simulink model "MyModel_Close_v1"  (R2018b)
settings: Solver=ode45  StartTime=0.0  StopTime=0.3  RelTol=1e-3
InitFcn:
  | tpwm = 0.0001;
  | K = 0.0604;
  | L1 = 0.00248;
  | L2 = -1.236e-7 * 40;
  | Td = 0;
  | kr = 50;
  | wc = 5;
  | speedref = 10;
  | L1 = 0.00248;
  | L2 = -1.239e-7 * 200;
libraries: powerlib x22, powerlib_meascontrol x12, powerlib_extras x5, simulink x2
settings Model: Creator=chenhao  LastModifiedBy=chenhao

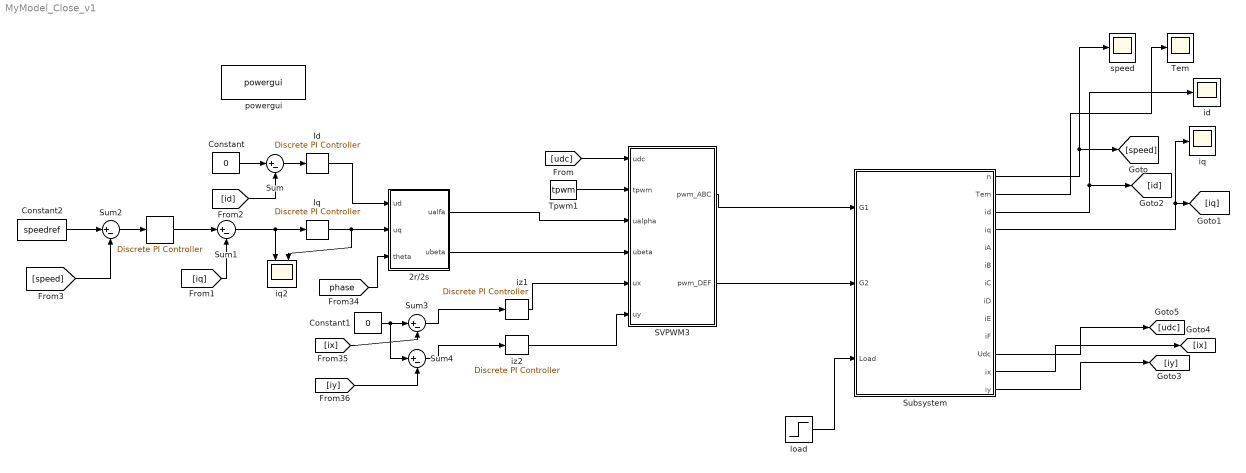
== system MyModel_Close_v1 ==
  "    " : powerlib_extras/Discrete  Control Blocks/Discrete PI Controller  Kp=1  Ki=80  Par_Limits=[50 -50]  Init=0  Ts=tpwm
  " Id" : powerlib_extras/Discrete  Control Blocks/Discrete PI Controller  Kp=3  Ki=120  Par_Limits=[300 -300]  Init=0  Ts=tpwm
  " Iq" : powerlib_extras/Discrete  Control Blocks/Discrete PI Controller  Kp=3  Ki=120  Par_Limits=[300 -300]  Init=0  Ts=tpwm
  " iz1" : powerlib_extras/Discrete  Control Blocks/Discrete PI Controller  Kp=10  Ki=100  Par_Limits=[300 -300]  Init=0  Ts=tpwm
  " iz2" : powerlib_extras/Discrete  Control Blocks/Discrete PI Controller  Kp=10  Ki=100  Par_Limits=[300 -300]  Init=0  Ts=tpwm
  2r/2s : Subsystem
  Constant : Constant  Value=0
  Constant1 : Constant  Value=0
  Constant2 : Constant  Value=speedref
  SVPWM3 : Subsystem
  Subsystem : Subsystem
  Sum{,1..4} (5 alike) : Sum  Inputs=|+-
  Tem : Scope
  Tpwm1 : Constant  Value=tpwm
  id : Scope
  iq : Scope
  iq2 : Scope  NumInputPorts=2
  load : Step  Time=0.1  After=5  SampleTime=0
  powergui : powerlib/powergui  Priority=1  SimulationMode=Discrete  SampleTime=5e-7  frequency=60  Iterations=50  frequencyindice=0  Pbase=100e6  ErrMax=1e-4  UnitsV=kV  UnitsW=MW  buscounter=0  FunctionMessages=off  echomessages=off  EnableUseOfTLC=off  CurrentSourceSwitches=off  DisableSnubberDevices=off  DisableRonSwitches=off  DisableVfSwitches=off  DisplayEquations=off  SolverType=Tustin  Interpol=off  ExternalGateDelay=off  methode=off  Ts=0  x0status=blocks  SPID=off  SwTol=0  HookPort=off  RestoreLinks=warning  ResistiveCurrentMeasurement=off  Frange=[0:2:500]  Ylog=off  Xlog=on  ShowGrid=off  save=off  variable=ZData  structure=Ia  ZoomFFT=on  StartTime=0.1  cycles=2  DisplayStyle=1  fundamental=2.5  FreqAxis=on  MaxFrequency=30  frequencyindicesteady=1  RmsSteady=1  display=off
  speed : Scope
  wires:
  SVPWM3/1(pwm_ABC) -> Subsystem/1(G1)
  " Iq"/1 -> iq2/2, 2r/2s/2(uq)
  " Id"/1 -> 2r/2s/1(ud)
  Sum/1 -> " Id"/1
  "    "/1 -> Sum1/1
  [id] -> Sum/2
  Sum1/1 -> iq2/1, " Iq"/1
  [iy] -> Sum4/2
  [speed] -> Sum2/2
  " iz2"/1 -> SVPWM3/6(uy)
  Tpwm1/1 -> SVPWM3/2(tpwm)
  [ix] -> Sum3/2
  Sum4/1 -> " iz2"/1
  Sum3/1 -> " iz1"/1
  Constant/1 -> Sum/1
  Sum2/1 -> "    "/1
  [phase] -> 2r/2s/3(theta)
  SVPWM3/2(pwm_DEF) -> Subsystem/2(G2)
  2r/2s/1(ualfa) -> SVPWM3/3(ualpha)
  [iq] -> Sum1/2
  2r/2s/2(ubeta) -> SVPWM3/4(ubeta)
  Constant1/1 -> Sum4/1, Sum3/1
  " iz1"/1 -> SVPWM3/5(ux)
  Constant2/1 -> Sum2/1
  Subsystem/1(n) -> speed/1, [speed]
  Subsystem/4(iq) -> iq/1, [iq]
  Subsystem/3(id) -> id/1, [id]
  Subsystem/12(ix) -> [ix]
  Subsystem/13("iy ") -> [iy]
  Subsystem/11(Udc) -> [udc]
  [udc] -> SVPWM3/1(udc)
  load/1 -> Subsystem/3(Load)
  Subsystem/2(Tem) -> Tem/1

== system MyModel_Close_v1/2r//2s ==
  ud : Inport
  uq : Inport  Port=2
  theta : Inport  Port=3
  Fcn : Fcn  Expr=u(1)*cos(u(3))-u(2)*sin(u(3))
  Fcn1 : Fcn  Expr=u(1)*sin(u(3))+u(2)*cos(u(3))
  Mux1 : Mux  Inputs=3
  ualfa : Outport
  ubeta : Outport  Port=2
  wires:
  theta/1 -> Mux1/3
  uq/1 -> Mux1/2
  ud/1 -> Mux1/1
  Fcn1/1 -> ubeta/1
  Fcn/1 -> ualfa/1
  Mux1/1 -> Fcn1/1, Fcn/1

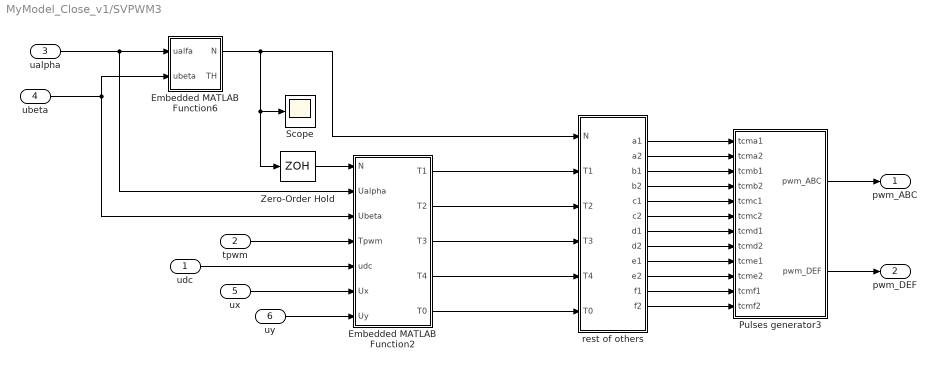
== system MyModel_Close_v1/SVPWM3 ==
  udc : Inport
  tpwm : Inport  Port=2
  ualpha : Inport  Port=3
  ubeta : Inport  Port=4
  ux : Inport  Port=5
  uy : Inport  Port=6
  Embedded MATLAB Function2 : MATLAB Function  TreatAsAtomicUnit=on
  Embedded MATLAB Function6 : MATLAB Function  TreatAsAtomicUnit=on
  Pulses generator3 : Subsystem
  Scope : Scope
  Zero-Order Hold : ZeroOrderHold  SampleTime=1e-4
  rest of others : MATLAB Function  TreatAsAtomicUnit=on
  pwm_ABC : Outport
  pwm_DEF : Outport  Port=2
  wires:
  udc/1 -> Embedded MATLAB Function2/5(udc)
  Embedded MATLAB Function2/4(T4) -> rest of others/5(T4)
  Embedded MATLAB Function2/1(T1) -> rest of others/2(T1)
  Pulses generator3/1(pwm_ABC) -> pwm_ABC/1
  Pulses generator3/2(pwm_DEF) -> pwm_DEF/1
  rest of others/12(f2) -> Pulses generator3/12(tcmf2)
  rest of others/11(f1) -> Pulses generator3/11(tcmf1)
  rest of others/10(e2) -> Pulses generator3/10(tcme2)
  rest of others/9(e1) -> Pulses generator3/9(tcme1)
  rest of others/8(d2) -> Pulses generator3/8(tcmd2)
  rest of others/7(d1) -> Pulses generator3/7(tcmd1)
  rest of others/6(c2) -> Pulses generator3/6(tcmc2)
  rest of others/5(c1) -> Pulses generator3/5(tcmc1)
  rest of others/4(b2) -> Pulses generator3/4(tcmb2)
  rest of others/3(b1) -> Pulses generator3/3(tcmb1)
  rest of others/2(a2) -> Pulses generator3/2(tcma2)
  rest of others/1(a1) -> Pulses generator3/1(tcma1)
  Embedded MATLAB Function2/2(T2) -> rest of others/3(T2)
  tpwm/1 -> Embedded MATLAB Function2/4(Tpwm)
  Embedded MATLAB Function2/5(T0) -> rest of others/6(T0)
  ualpha/1 -> Embedded MATLAB Function2/2(Ualpha), Embedded MATLAB Function6/1(ualfa)
  ubeta/1 -> Embedded MATLAB Function6/2(ubeta), Embedded MATLAB Function2/3(Ubeta)
  ux/1 -> Embedded MATLAB Function2/6(Ux)
  uy/1 -> Embedded MATLAB Function2/7(Uy)
  Embedded MATLAB Function2/3(T3) -> rest of others/4(T3)
  Zero-Order Hold/1 -> Embedded MATLAB Function2/1(N)
  Embedded MATLAB Function6/1(N) -> rest of others/1(N), Scope/1, Zero-Order Hold/1

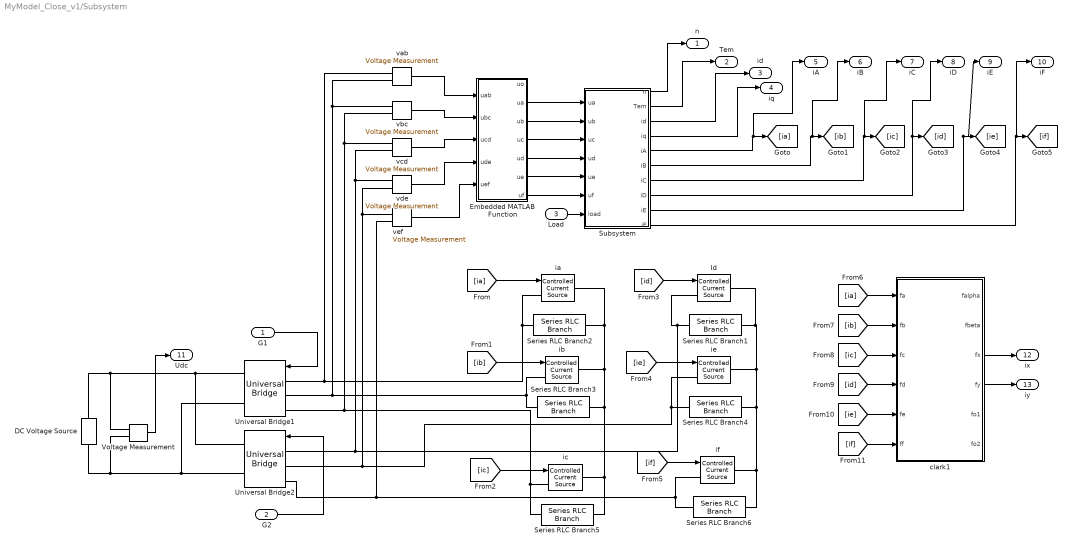
== system MyModel_Close_v1/Subsystem ==
  G1 : Inport
  G2 : Inport  Port=2
  Load : Inport  Port=3
  DC Voltage Source : powerlib/Electrical Sources/DC Voltage Source  Amplitude=100  Measurements=Voltage
  Embedded MATLAB Function : MATLAB Function  TreatAsAtomicUnit=on
  Id : powerlib/Electrical Sources/Controlled Current Source  Initialize=on  Source_Type=AC  Amplitude=0  Phase=0  Frequency=0  Measurements=None
  Series RLC Branch{1..6} (6 alike) : powerlib/Elements/Series RLC Branch  LConnTagsString=__new0  RConnTagsString=__new0  BranchType=R  Resistance=10e10  Inductance=10e-7  SetiL0=off  InitialCurrent=0  Capacitance=1e-6  Setx0=off  InitialVoltage=0  Measurements=None
  Subsystem : Subsystem
  Universal Bridge1 : powerlib/Power Electronics/Universal Bridge  Arms=3  SnubberResistance=1e5  SnubberCapacitance=inf  Device=IGBT / Diodes  Ron=1e-3  Lon=0  ForwardVoltages="[  0  0  ]"  ForwardVoltage=0  GTOparameters=[ 10e-6 , 20e-6 ]  IGBTparameters=[ 0 , 0 ]  Measurements=None  Measurements_2=None  converterType=Rectifier
  Universal Bridge2 : powerlib/Power Electronics/Universal Bridge  Arms=3  SnubberResistance=1e5  SnubberCapacitance=inf  Device=IGBT / Diodes  Ron=1e-3  Lon=0  ForwardVoltages="[  0  0  ]"  ForwardVoltage=0  GTOparameters=[ 10e-6 , 20e-6 ]  IGBTparameters=[ 0 , 0 ]  Measurements=None  Measurements_2=None  converterType=Rectifier
  Voltage Measurement : powerlib/Measurements/Voltage Measurement  PhasorSimulation=off  OutputType=Complex  PSBequivalent=0
  clark1 : MATLAB Function  TreatAsAtomicUnit=on
  ia : powerlib/Electrical Sources/Controlled Current Source  Initialize=on  Source_Type=AC  Amplitude=0  Phase=0  Frequency=0  Measurements=None
  ib : powerlib/Electrical Sources/Controlled Current Source  Initialize=on  Source_Type=AC  Amplitude=0  Phase=0  Frequency=0  Measurements=None
  ic : powerlib/Electrical Sources/Controlled Current Source  Initialize=on  Source_Type=AC  Amplitude=0  Phase=0  Frequency=0  Measurements=None
  ie : powerlib/Electrical Sources/Controlled Current Source  Initialize=on  Source_Type=AC  Amplitude=0  Phase=0  Frequency=0  Measurements=None
  if : powerlib/Electrical Sources/Controlled Current Source  Initialize=on  Source_Type=AC  Amplitude=0  Phase=0  Frequency=0  Measurements=None
  "vab " : powerlib/Measurements/Voltage Measurement  PhasorSimulation=off  OutputType=Complex  PSBequivalent=0
  vbc : powerlib/Measurements/Voltage Measurement  PhasorSimulation=off  OutputType=Complex  PSBequivalent=0
  vcd : powerlib/Measurements/Voltage Measurement  PhasorSimulation=off  OutputType=Complex  PSBequivalent=0
  vde : powerlib/Measurements/Voltage Measurement  PhasorSimulation=off  OutputType=Complex  PSBequivalent=0
  vef : powerlib/Measurements/Voltage Measurement  PhasorSimulation=off  OutputType=Complex  PSBequivalent=0
  n : Outport
  Tem : Outport  Port=2
  id : Outport  Port=3
  iq : Outport  Port=4
  iA : Outport  Port=5
  iB : Outport  Port=6
  iC : Outport  Port=7
  iD : Outport  Port=8
  iE : Outport  Port=9
  iF : Outport  Port=10
  Udc : Outport  Port=11
  ix : Outport  Port=12
  "iy " : Outport  Port=13
  wires:
  G1/1 -> Universal Bridge1/1
  G2/1 -> Universal Bridge2/1
  Voltage Measurement/1 -> Udc/1
  "vab "/1 -> Embedded MATLAB Function/1(uab)
  vbc/1 -> Embedded MATLAB Function/2(ubc)
  vcd/1 -> Embedded MATLAB Function/3(ucd)
  vde/1 -> Embedded MATLAB Function/4(ude)
  vef/1 -> Embedded MATLAB Function/5(uef)
  [ia] -> ia/1
  [ib] -> ib/1
  [ic] -> ic/1
  [id] -> Id/1
  [ie] -> ie/1
  [if] -> if/1
  [ia] -> clark1/1(fa)
  [ib] -> clark1/2(fb)
  [ic] -> clark1/3(fc)
  [id] -> clark1/4(fd)
  [ie] -> clark1/5(fe)
  [if] -> clark1/6(ff)
  clark1/3(fx) -> ix/1
  clark1/4(fy) -> "iy "/1
  Embedded MATLAB Function/6(ue) -> Subsystem/5(ue)
  Embedded MATLAB Function/2(ua) -> Subsystem/1(ua)
  Embedded MATLAB Function/3(ub) -> Subsystem/2(ub)
  Embedded MATLAB Function/4(uc) -> Subsystem/3(uc)
  Embedded MATLAB Function/5(ud) -> Subsystem/4(ud)
  Embedded MATLAB Function/7(uf) -> Subsystem/6(uf)
  Load/1 -> Subsystem/7(load)
  Subsystem/1(n) -> n/1
  Subsystem/2(Tem) -> Tem/1
  Subsystem/3(id) -> id/1
  Subsystem/4(iq) -> iq/1
  Subsystem/5(iA) -> iA/1, [ia]
  Subsystem/6(iB) -> iB/1, [ib]
  Subsystem/7(iC) -> iC/1, [ic]
  Subsystem/8(iD) -> iD/1, [id]
  Subsystem/9(iE) -> iE/1, [ie]
  Subsystem/10(iF) -> iF/1, [if]
  connections:
  Series RLC Branch4/LConn1 -- vef/LConn1 -- vde/LConn2 -- Universal Bridge2/LConn2 -- ie/LConn1
  Series RLC Branch6/LConn1 -- vef/LConn2 -- Universal Bridge2/LConn3 -- if/LConn1
  Universal Bridge1/RConn2 -- DC Voltage Source/LConn1 -- Voltage Measurement/LConn2 -- Universal Bridge2/RConn2
  DC Voltage Source/RConn1 -- Voltage Measurement/LConn1 -- Universal Bridge2/RConn1 -- Universal Bridge1/RConn1
  ia/LConn1 -- "vab "/LConn1 -- Universal Bridge1/LConn1 -- Series RLC Branch2/LConn1
  ib/LConn1 -- vbc/LConn1 -- "vab "/LConn2 -- Universal Bridge1/LConn2 -- Series RLC Branch3/LConn1
  ic/LConn1 -- vcd/LConn1 -- vbc/LConn2 -- Universal Bridge1/LConn3 -- Series RLC Branch5/LConn1
  Series RLC Branch2/RConn1 -- ia/RConn1 -- ib/RConn1 -- Series RLC Branch3/RConn1 -- ic/RConn1 -- Series RLC Branch5/RConn1
  Series RLC Branch1/RConn1 -- Id/RConn1 -- ie/RConn1 -- Series RLC Branch4/RConn1 -- if/RConn1 -- Series RLC Branch6/RConn1
  Universal Bridge2/LConn1 -- vde/LConn1 -- vcd/LConn2 -- Id/LConn1 -- Series RLC Branch1/LConn1

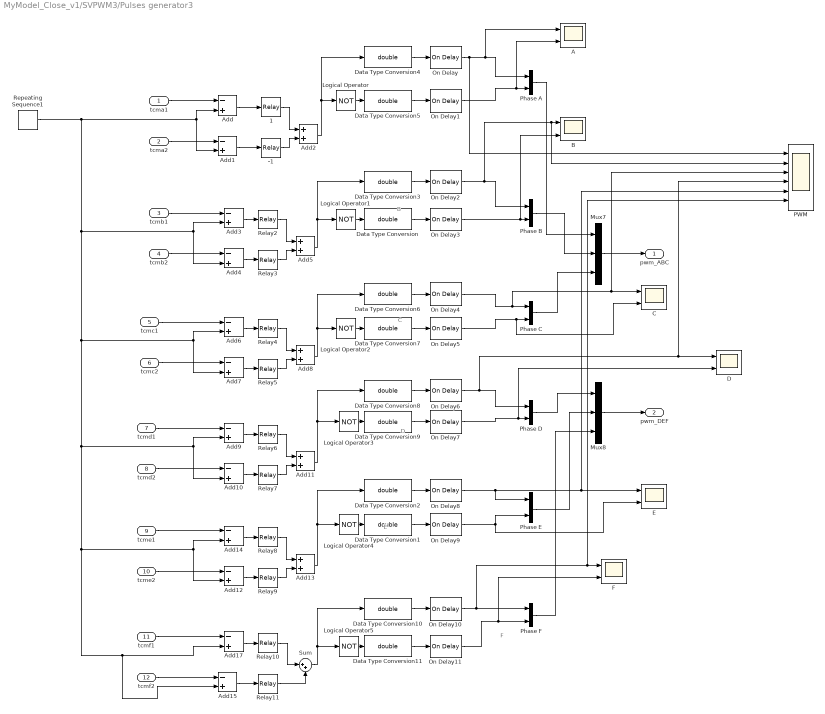
== system MyModel_Close_v1/SVPWM3/Pulses generator3 ==
  note: B
  note: C
  note: D
  note: E
  note: F
  tcma1 : Inport
  tcma2 : Inport  Port=2
  tcmb1 : Inport  Port=3
  tcmb2 : Inport  Port=4
  tcmc1 : Inport  Port=5
  tcmc2 : Inport  Port=6
  tcmd1 : Inport  Port=7
  tcmd2 : Inport  Port=8
  tcme1 : Inport  Port=9
  tcme2 : Inport  Port=10
  tcmf1 : Inport  Port=11
  tcmf2 : Inport  Port=12
  -1 : Relay  OnOutputValue=-1
  1 : Relay
  A : Scope  NumInputPorts=2
  Add{,1,3..4,6..7,9..10,12,14..15,17} (12 alike) : Sum  Inputs=-+
  Add{2,5,8,11,13} (5 alike) : Sum
  B : Scope  NumInputPorts=2
  C : Scope  NumInputPorts=2
  D : Scope  NumInputPorts=2
  Data Type Conversion{,1..11} (12 alike) : DataTypeConversion  OutDataTypeStr=double
  E : Scope  NumInputPorts=2
  F : Scope  NumInputPorts=2
  Logical Operator{,1..5} (6 alike) : Logic  Operator=NOT  AllPortsSameDT=off  OutDataTypeStr=boolean
  Mux7 : Mux  Inputs=3
  Mux8 : Mux  Inputs=3
  On Delay{,1..11} (12 alike) : powerlib_meascontrol/Logic/On Delay  DelayType=On delay  delay=Td  ic=0  Ts=0
      settings: SourceProductName=Simscape Power Systems
  PWM : Scope  NumInputPorts=6
  Phase A : Mux  Inputs=2
  Phase B : Mux  Inputs=2
  Phase C : Mux  Inputs=2
  Phase D : Mux  Inputs=2
  Phase E : Mux  Inputs=2
  Phase F : Mux  Inputs=2
  Relay{2,4,6,8,10} (5 alike) : Relay
  Relay{3,5,7,9,11} (5 alike) : Relay  OnOutputValue=-1
  Repeating Sequence1 : simulink/Sources/Repeating Sequence  rep_seq_t=[0 tpwm]  rep_seq_y=[0 tpwm]
  Sum : Sum  Inputs=|++
  pwm_ABC : Outport
  pwm_DEF : Outport  Port=2
  wires:
  On Delay11/1 -> F/2, Phase F/2
  Data Type Conversion11/1 -> On Delay11/1
  On Delay10/1 -> PWM/6, F/1, Phase F/1
  Data Type Conversion10/1 -> On Delay10/1
  On Delay9/1 -> E/2, Phase E/2
  Data Type Conversion1/1 -> On Delay9/1
  On Delay8/1 -> Phase E/1, PWM/5, E/1
  Data Type Conversion2/1 -> On Delay8/1
  On Delay7/1 -> D/2, Phase D/2
  Data Type Conversion9/1 -> On Delay7/1
  On Delay6/1 -> PWM/4, D/1, Phase D/1
  Data Type Conversion8/1 -> On Delay6/1
  On Delay5/1 -> C/2, Phase C/2
  Data Type Conversion7/1 -> On Delay5/1
  On Delay4/1 -> PWM/3, C/1, Phase C/1
  Data Type Conversion6/1 -> On Delay4/1
  On Delay2/1 -> PWM/2, B/1, Phase B/1
  On Delay3/1 -> B/2, Phase B/2
  Data Type Conversion/1 -> On Delay3/1
  Data Type Conversion3/1 -> On Delay2/1
  On Delay1/1 -> A/2, Phase A/2
  Data Type Conversion5/1 -> On Delay1/1
  On Delay/1 -> A/1, Phase A/1, PWM/1
  Data Type Conversion4/1 -> On Delay/1
  Logical Operator3/1 -> Data Type Conversion9/1
  Logical Operator2/1 -> Data Type Conversion7/1
  Logical Operator/1 -> Data Type Conversion5/1
  Logical Operator1/1 -> Data Type Conversion/1
  Logical Operator4/1 -> Data Type Conversion1/1
  Add5/1 -> Logical Operator1/1, Data Type Conversion3/1
  Add2/1 -> Logical Operator/1, Data Type Conversion4/1
  Mux8/1 -> pwm_DEF/1
  Mux7/1 -> pwm_ABC/1
  Sum/1 -> Logical Operator5/1, Data Type Conversion10/1
  Add13/1 -> Logical Operator4/1, Data Type Conversion2/1
  Add11/1 -> Logical Operator3/1, Data Type Conversion8/1
  Add8/1 -> Logical Operator2/1, Data Type Conversion6/1
  Logical Operator5/1 -> Data Type Conversion11/1
  tcmf2/1 -> Add15/1
  Relay11/1 -> Sum/2
  Relay10/1 -> Sum/1
  Add17/1 -> Relay10/1
  tcmf1/1 -> Add17/1
  tcme2/1 -> Add12/1
  Relay9/1 -> Add13/2
  Relay8/1 -> Add13/1
  Add12/1 -> Relay9/1
  Add14/1 -> Relay8/1
  tcme1/1 -> Add14/1
  tcmd2/1 -> Add10/1
  Relay7/1 -> Add11/2
  Relay6/1 -> Add11/1
  Add10/1 -> Relay7/1
  Add9/1 -> Relay6/1
  tcmd1/1 -> Add9/1
  tcmc2/1 -> Add7/1
  Relay5/1 -> Add8/2
  Relay4/1 -> Add8/1
  Add7/1 -> Relay5/1
  Add6/1 -> Relay4/1
  tcmb2/1 -> Add4/1
  Relay3/1 -> Add5/2
  Relay2/1 -> Add5/1
  Add4/1 -> Relay3/1
  Add3/1 -> Relay2/1
  tcma1/1 -> Add/1
  -1/1 -> Add2/2
  1/1 -> Add2/1
  Add1/1 -> -1/1
  Add/1 -> 1/1
  Repeating Sequence1/1 -> Add15/2, Add17/2, Add12/2, Add14/2, Add9/2, Add10/2, Add7/2, Add6/2, Add3/2, Add4/2, Add1/2, Add/2
  tcma2/1 -> Add1/1
  tcmb1/1 -> Add3/1
  tcmc1/1 -> Add6/1
  Add15/1 -> Relay11/1
  Phase A/1 -> Mux7/1
  Phase B/1 -> Mux7/2
  Phase C/1 -> Mux7/3
  Phase D/1 -> Mux8/1
  Phase E/1 -> Mux8/2
  Phase F/1 -> Mux8/3

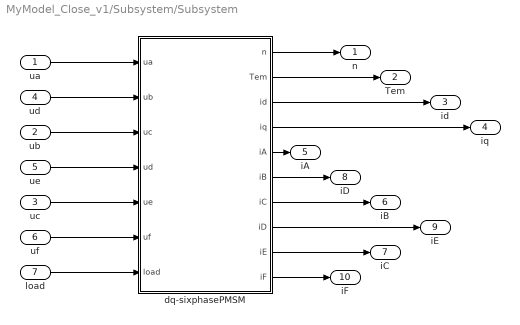
== system MyModel_Close_v1/Subsystem/Subsystem ==
  ua : Inport
  ub : Inport  Port=2
  uc : Inport  Port=3
  ud : Inport  Port=4
  ue : Inport  Port=5
  uf : Inport  Port=6
  load : Inport  Port=7
  dq-sixphasePMSM : Subsystem  mask{R=0.099, Ld=2.463342136542000e-03, Lq=2.473254136542000e-03, Lf=1.520747e-3, psi=0.0592, p=5, J=0.00174}
      mask prompts: R "Resistance (Om)"; Ld "d-inductance (H)"; Lq "q-inductance (H)"; Lf "Leak inductance (H)"; psi "flux (Wb)"; p "pole pairs"; J "inertia (kg*m^2)"
  n : Outport
  Tem : Outport  Port=2
  id : Outport  Port=3
  iq : Outport  Port=4
  iA : Outport  Port=5
  iB : Outport  Port=6
  iC : Outport  Port=7
  iD : Outport  Port=8
  iE : Outport  Port=9
  iF : Outport  Port=10
  wires:
  ua/1 -> dq-sixphasePMSM/1(ua)
  ub/1 -> dq-sixphasePMSM/3(uc)
  uc/1 -> dq-sixphasePMSM/5(ue)
  ud/1 -> dq-sixphasePMSM/2(ub)
  ue/1 -> dq-sixphasePMSM/4(ud)
  uf/1 -> dq-sixphasePMSM/6(uf)
  load/1 -> dq-sixphasePMSM/7(load)
  dq-sixphasePMSM/1(n) -> n/1
  dq-sixphasePMSM/2(Tem) -> Tem/1
  dq-sixphasePMSM/3(id) -> id/1
  dq-sixphasePMSM/4(iq) -> iq/1
  dq-sixphasePMSM/5(iA) -> iA/1
  dq-sixphasePMSM/6(iB) -> iD/1
  dq-sixphasePMSM/7(iC) -> iB/1
  dq-sixphasePMSM/8(iD) -> iE/1
  dq-sixphasePMSM/9(iE) -> iC/1
  dq-sixphasePMSM/10(iF) -> iF/1

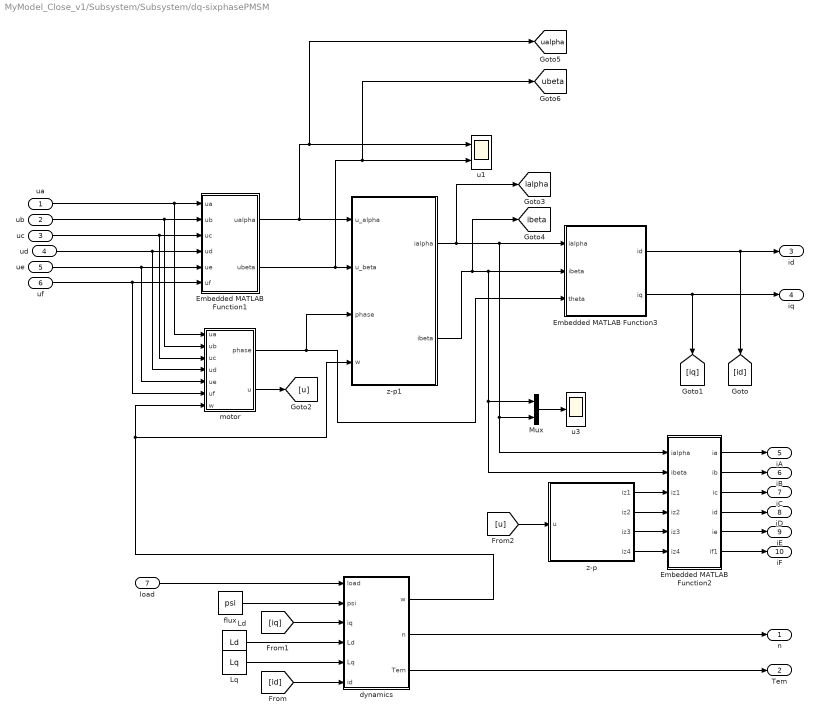
== system MyModel_Close_v1/Subsystem/Subsystem/dq-sixphasePMSM ==
  ua : Inport
  ub : Inport  Port=2
  uc : Inport  Port=3
  ud : Inport  Port=4
  ue : Inport  Port=5
  uf : Inport  Port=6
  load : Inport  Port=7
  Embedded MATLAB Function1 : MATLAB Function  TreatAsAtomicUnit=on
  Embedded MATLAB Function2 : MATLAB Function  TreatAsAtomicUnit=on
  Embedded MATLAB Function3 : MATLAB Function  TreatAsAtomicUnit=on
  Ld : Constant  Value=Ld
  Lq : Constant  Value=Lq
  Mux : Mux  Inputs=2
  dynamics : Subsystem
  flux : Constant  Value=psi
  motor : Subsystem
  u1 : Scope  NumInputPorts=2
  u3 : Scope
  z-p : Subsystem
  z-p1 : Subsystem
  n : Outport
  Tem : Outport  Port=2
  id : Outport  Port=3
  iq : Outport  Port=4
  iA : Outport  Port=5
  iB : Outport  Port=6
  iC : Outport  Port=7
  iD : Outport  Port=8
  iE : Outport  Port=9
  iF : Outport  Port=10
  tag scope: ialpha=global, ibeta=global, ualpha=global, ubeta=global
  wires:
  Embedded MATLAB Function2/3(ic) -> iC/1
  Embedded MATLAB Function2/5(ie) -> iE/1
  Embedded MATLAB Function2/4(id) -> iD/1
  Embedded MATLAB Function2/1(ia) -> iA/1
  Embedded MATLAB Function2/2(ib) -> iB/1
  Embedded MATLAB Function2/6(if1) -> iF/1
  ua/1 -> motor/1(ua), Embedded MATLAB Function1/1(ua)
  uc/1 -> motor/3(uc), Embedded MATLAB Function1/3(uc)
  ud/1 -> motor/4(ud), Embedded MATLAB Function1/4(ud)
  ue/1 -> motor/5(ue), Embedded MATLAB Function1/5(ue)
  uf/1 -> motor/6(uf), Embedded MATLAB Function1/6(uf)
  Ld/1 -> dynamics/4(Ld)
  Lq/1 -> dynamics/5(Lq)
  load/1 -> dynamics/1(load)
  flux/1 -> dynamics/2(psi)
  [id] -> dynamics/6(id)
  [iq] -> dynamics/3(iq)
  z-p/2(iz2) -> Embedded MATLAB Function2/4(iz2)
  z-p/1(iz1) -> Embedded MATLAB Function2/3(iz1)
  z-p/4(iz4) -> Embedded MATLAB Function2/6(iz4)
  z-p/3(iz3) -> Embedded MATLAB Function2/5(iz3)
  ub/1 -> motor/2(ub), Embedded MATLAB Function1/2(ub)
  [u] -> z-p/1(u)
  z-p1/1(ialpha) -> [ialpha], Mux/2, Embedded MATLAB Function2/1(ialpha), Embedded MATLAB Function3/1(ialpha)
  z-p1/2(ibeta) -> [ibeta], Mux/1, Embedded MATLAB Function2/2(ibeta), Embedded MATLAB Function3/2(ibeta)
  Embedded MATLAB Function3/1(id) -> [id], id/1
  Embedded MATLAB Function3/2(iq) -> iq/1, [iq]
  Mux/1 -> u3/1
  dynamics/1(w) -> z-p1/4(w), motor/7(w)
  dynamics/2(n) -> n/1
  dynamics/3(Tem) -> Tem/1
  motor/2(u) -> [u]
  motor/1(phase) -> Embedded MATLAB Function3/3(theta), z-p1/3(phase)
  Embedded MATLAB Function1/1(ualpha) -> [ualpha], u1/1, z-p1/1(u_alpha)
  Embedded MATLAB Function1/2(ubeta) -> [ubeta], u1/2, z-p1/2(u_beta)

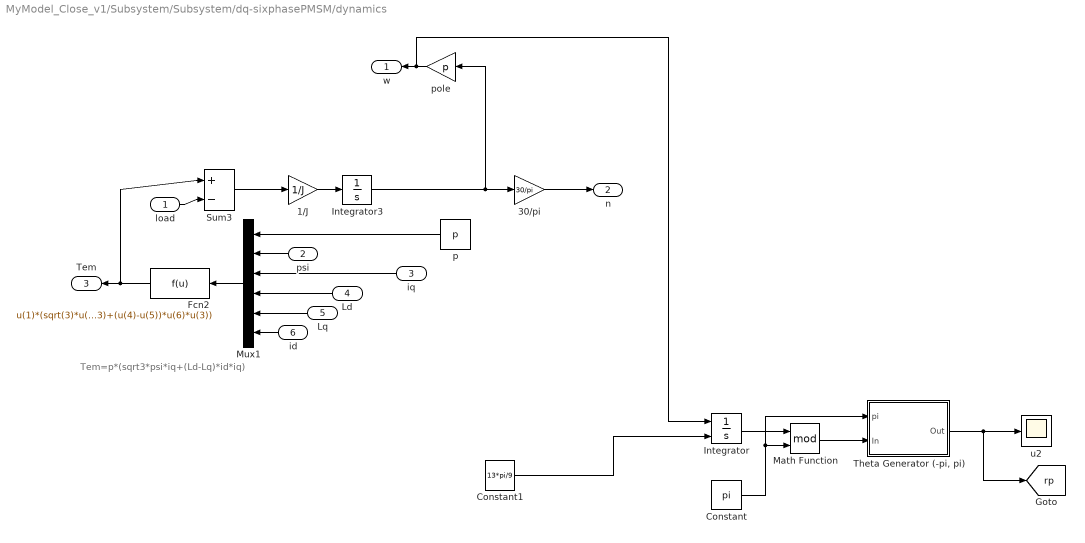
== system MyModel_Close_v1/Subsystem/Subsystem/dq-sixphasePMSM/dynamics ==
  note: Tem=p*(sqrt3*psi*iq+(Ld-Lq)*id*iq)
  load : Inport
  psi : Inport  Port=2
  iq : Inport  Port=3
  Ld : Inport  Port=4
  Lq : Inport  Port=5
  id : Inport  Port=6
  1/J : Gain  Gain=1/J  SaturateOnIntegerOverflow=on  OutDataTypeStr=Inherit: Same as input  ParamDataTypeStr=Inherit: Same as input
  30/pi : Gain  Gain=30/pi  SaturateOnIntegerOverflow=on  OutDataTypeStr=Inherit: Same as input  ParamDataTypeStr=Inherit: Same as input
  Constant : Constant  Value=pi
  Constant1 : Constant  Value=13*pi/9
  Fcn2 : Fcn  Expr=u(1)*(sqrt(3)*u(2)*u(3)+(u(4)-u(5))*u(6)*u(3))
  Integrator : Integrator  InitialConditionSource=external
  Integrator3 : Integrator
  Math Function : Math  Operator=mod  SaturateOnIntegerOverflow=on
  Mux1 : Mux  Inputs=6
  Sum3 : Sum  Inputs=|+-  SaturateOnIntegerOverflow=on
  "Theta Generator (-pi, pi)" : Subsystem
  p : Constant  Value=p
  pole : Gain  Gain=p  SaturateOnIntegerOverflow=on  OutDataTypeStr=Inherit: Same as input  ParamDataTypeStr=Inherit: Same as input
  u2 : Scope
  w : Outport
  n : Outport  Port=2
  Tem : Outport  Port=3
  tag scope: rp=global
  wires:
  p/1 -> Mux1/1
  Mux1/1 -> Fcn2/1
  Fcn2/1 -> Sum3/1, Tem/1
  Sum3/1 -> 1/J/1
  1/J/1 -> Integrator3/1
  Integrator3/1 -> 30/pi/1, pole/1
  psi/1 -> Mux1/2
  Ld/1 -> Mux1/4
  Lq/1 -> Mux1/5
  30/pi/1 -> n/1
  load/1 -> Sum3/2
  iq/1 -> Mux1/3
  id/1 -> Mux1/6
  pole/1 -> Integrator/1, w/1
  Integrator/1 -> Math Function/1
  Constant/1 -> Math Function/2, "Theta Generator (-pi, pi)"/1(pi)
  Math Function/1 -> "Theta Generator (-pi, pi)"/2(In)
  Constant1/1 -> Integrator/2
  "Theta Generator (-pi, pi)"/1(Out) -> [rp], u2/1

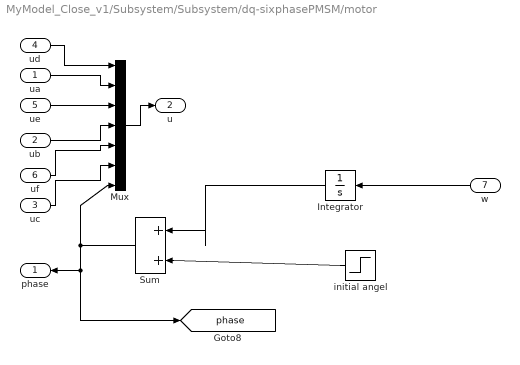
== system MyModel_Close_v1/Subsystem/Subsystem/dq-sixphasePMSM/motor ==
  ua : Inport
  ub : Inport  Port=2
  uc : Inport  Port=3
  ud : Inport  Port=4
  ue : Inport  Port=5
  uf : Inport  Port=6
  w : Inport  Port=7
  Integrator : Integrator
  Mux : Mux  Inputs=7
  Sum : Sum  Inputs=|++  SaturateOnIntegerOverflow=on
  initial angel : Step  Time=0  After=13*pi/9  SampleTime=0
  phase : Outport
  u : Outport  Port=2
  tag scope: phase=global
  wires:
  Sum/1 -> [phase], phase/1, Mux/7
  Integrator/1 -> Sum/1
  w/1 -> Integrator/1
  Mux/1 -> u/1
  ud/1 -> Mux/1
  ua/1 -> Mux/2
  ue/1 -> Mux/3
  ub/1 -> Mux/4
  uf/1 -> Mux/5
  uc/1 -> Mux/6
  initial angel/1 -> Sum/2

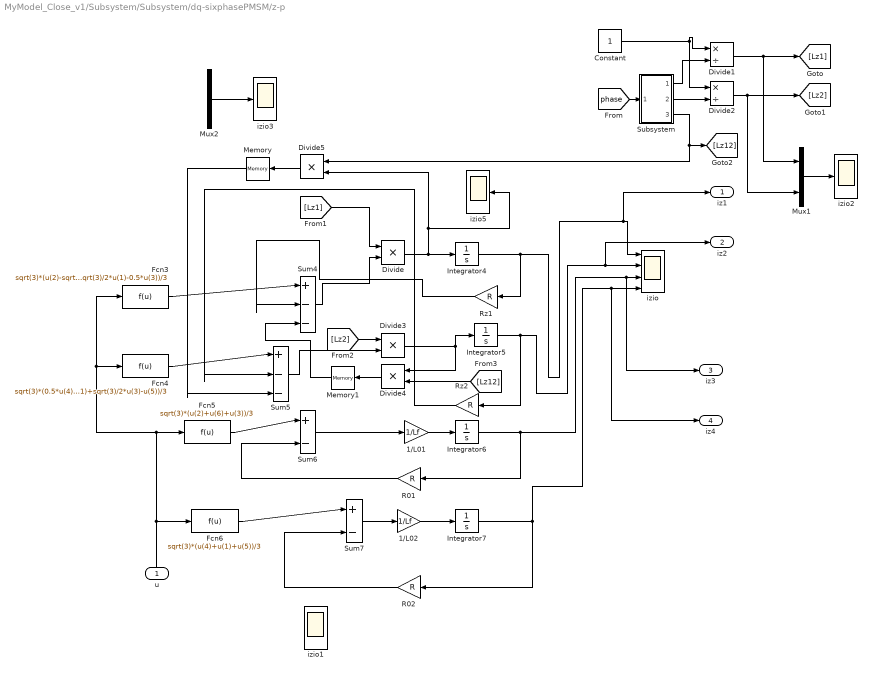
== system MyModel_Close_v1/Subsystem/Subsystem/dq-sixphasePMSM/z-p ==
  u : Inport
  1/L01 : Gain  Gain=1/Lf  SaturateOnIntegerOverflow=on  OutDataTypeStr=Inherit: Same as input  ParamDataTypeStr=Inherit: Same as input
  1/L02 : Gain  Gain=1/Lf  SaturateOnIntegerOverflow=on  OutDataTypeStr=Inherit: Same as input  ParamDataTypeStr=Inherit: Same as input
  Constant : Constant
  Divide{,3..5} (4 alike) : Product  Inputs=**
  Divide1 : Product  Inputs=*/
  Divide2 : Product  Inputs=*/
  Fcn3 : Fcn  Expr=sqrt(3)*(u(2)-sqrt(3)/2*u(4)-0.5*u(6)+sqrt(3)/2*u(1)-0.5*u(3))/3
  Fcn4 : Fcn  Expr=sqrt(3)*(0.5*u(4)-sqrt(3)/2*u(6)+0.5*u(1)+sqrt(3)/2*u(3)-u(5))/3
  Fcn5 : Fcn  Expr=sqrt(3)*(u(2)+u(6)+u(3))/3
  Fcn6 : Fcn  Expr=sqrt(3)*(u(4)+u(1)+u(5))/3
  Integrator{4..7} (4 alike) : Integrator
  Memory : Memory
  Memory1 : Memory
  Mux1 : Mux  Inputs=2
  Mux2 : Mux  Inputs=2
  R01 : Gain  Gain=R  SaturateOnIntegerOverflow=on  OutDataTypeStr=Inherit: Same as input  ParamDataTypeStr=Inherit: Same as input
  R02 : Gain  Gain=R  SaturateOnIntegerOverflow=on  OutDataTypeStr=Inherit: Same as input  ParamDataTypeStr=Inherit: Same as input
  Rz1 : Gain  Gain=R  SaturateOnIntegerOverflow=on  OutDataTypeStr=Inherit: Same as input  ParamDataTypeStr=Inherit: Same as input
  Rz2 : Gain  Gain=R  SaturateOnIntegerOverflow=on  OutDataTypeStr=Inherit: Same as input  ParamDataTypeStr=Inherit: Same as input
  Subsystem : Subsystem
  Sum4 : Sum  Inputs=|+--  SaturateOnIntegerOverflow=on
  Sum5 : Sum  Inputs=|+--  SaturateOnIntegerOverflow=on
  Sum6 : Sum  Inputs=|+-  SaturateOnIntegerOverflow=on
  Sum7 : Sum  Inputs=|+-  SaturateOnIntegerOverflow=on
  izio : Scope  NumInputPorts=4
  izio1 : Scope  NumInputPorts=4
  izio2 : Scope
  izio3 : Scope
  izio5 : Scope
  iz1 : Outport
  iz2 : Outport  Port=2
  iz3 : Outport  Port=3
  iz4 : Outport  Port=4
  wires:
  R02/1 -> Sum7/2
  R01/1 -> Sum6/2
  Rz2/1 -> Sum5/2
  Rz1/1 -> Sum4/2
  Integrator7/1 -> iz4/1, izio/4, R02/1
  1/L02/1 -> Integrator7/1
  Sum7/1 -> 1/L02/1
  Integrator6/1 -> iz3/1, izio/3, R01/1
  1/L01/1 -> Integrator6/1
  Sum6/1 -> 1/L01/1
  u/1 -> Fcn3/1, Fcn4/1, Fcn5/1, Fcn6/1
  [phase] -> Subsystem/1(Phase)
  Subsystem/1(Lz1) -> Divide1/2
  Divide1/1 -> Mux1/1, [Lz1]
  Constant/1 -> Divide1/1, Divide2/1
  Subsystem/2(Lz2) -> Divide2/2
  Divide2/1 -> Mux1/2, [Lz2]
  Mux1/1 -> izio2/1
  Sum4/1 -> Divide/2
  [Lz1] -> Divide/1
  Divide/1 -> izio5/1, Divide5/2, Integrator4/1
  Divide3/1 -> Integrator5/1, Divide4/1
  Sum5/1 -> Divide3/2
  [Lz2] -> Divide3/1
  Fcn5/1 -> Sum6/1
  Integrator5/1 -> Rz2/1, iz2/1, izio/2
  Integrator4/1 -> Rz1/1, iz1/1, izio/1
  Fcn4/1 -> Sum5/1
  Subsystem/3(Lz1z2) -> Divide5/1, [Lz12]
  Divide4/1 -> Memory1/1
  [Lz12] -> Divide4/2
  Divide5/1 -> Memory/1
  Memory1/1 -> Sum4/3
  Fcn6/1 -> Sum7/1
  Mux2/1 -> izio3/1
  Fcn3/1 -> Sum4/1
  Memory/1 -> Sum5/3

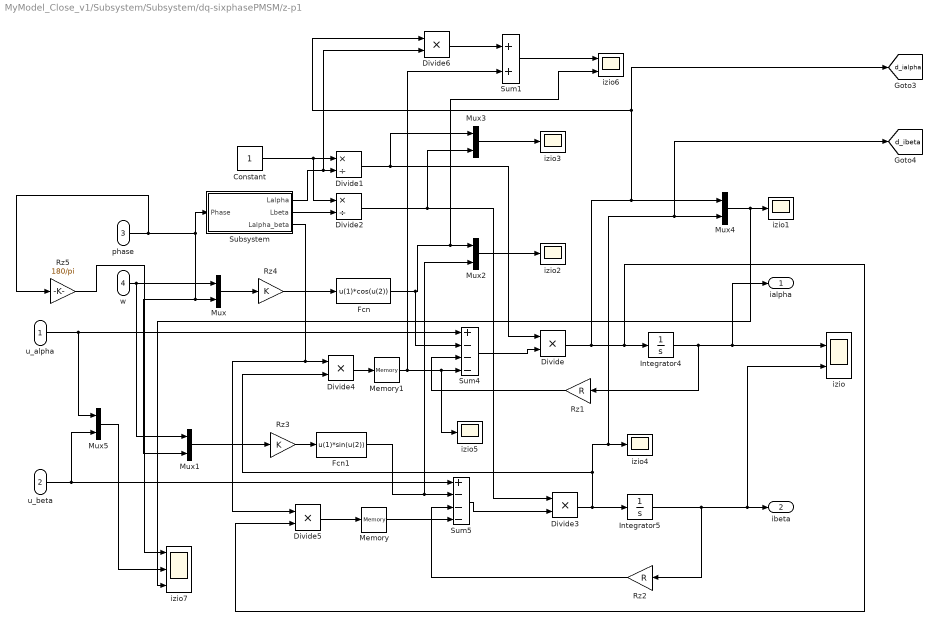
== system MyModel_Close_v1/Subsystem/Subsystem/dq-sixphasePMSM/z-p1 ==
  u_alpha : Inport
  u_beta : Inport  Port=2
  phase : Inport  Port=3
  w : Inport  Port=4
  Constant : Constant
  Divide{,3..6} (5 alike) : Product  Inputs=**
  Divide1 : Product  Inputs=*/
  Divide2 : Product  Inputs=*/
  Fcn : Fcn  Expr=u(1)*cos(u(2))
  Fcn1 : Fcn  Expr=u(1)*sin(u(2))
  Integrator4 : Integrator
  Integrator5 : Integrator
  Memory : Memory
  Memory1 : Memory
  Mux{,1..5} (6 alike) : Mux  Inputs=2
  Rz1 : Gain  Gain=R  SaturateOnIntegerOverflow=on  OutDataTypeStr=Inherit: Same as input  ParamDataTypeStr=Inherit: Same as input
  Rz2 : Gain  Gain=R  SaturateOnIntegerOverflow=on  OutDataTypeStr=Inherit: Same as input  ParamDataTypeStr=Inherit: Same as input
  Rz3 : Gain  Gain=K  SaturateOnIntegerOverflow=on  OutDataTypeStr=Inherit: Same as input  ParamDataTypeStr=Inherit: Same as input
  Rz4 : Gain  Gain=K  SaturateOnIntegerOverflow=on  OutDataTypeStr=Inherit: Same as input  ParamDataTypeStr=Inherit: Same as input
  Rz5 : Gain  Gain=180/pi  SaturateOnIntegerOverflow=on  OutDataTypeStr=Inherit: Same as input  ParamDataTypeStr=Inherit: Same as input
  Subsystem : Subsystem
  Sum1 : Sum  SaturateOnIntegerOverflow=on
  Sum4 : Sum  Inputs=+---  SaturateOnIntegerOverflow=on
  Sum5 : Sum  Inputs=+---  SaturateOnIntegerOverflow=on
  izio : Scope  NumInputPorts=2
  izio{1..5} (5 alike) : Scope
  izio6 : Scope  NumInputPorts=2
  izio7 : Scope  NumInputPorts=3
  ialpha : Outport
  ibeta : Outport  Port=2
  tag scope: d_ialpha=global, d_ibeta=global
  wires:
  phase/1 -> Rz5/1, Subsystem/1(Phase), Mux1/2, Mux/2
  Subsystem/1(Lalpha) -> Divide6/2, Divide1/2
  Constant/1 -> Divide1/1, Divide2/1
  Subsystem/2(Lbeta) -> Divide2/2
  Sum4/1 -> Divide/2
  Divide/1 -> Divide6/1, [d_ialpha], Mux4/1, Divide5/2, Integrator4/1
  Divide3/1 -> [d_ibeta], Mux4/2, izio4/1, Divide4/2, Integrator5/1
  Sum5/1 -> Divide3/2
  Integrator4/1 -> Rz1/1, ialpha/1, izio/1
  Rz1/1 -> Sum4/3
  Rz2/1 -> Sum5/3
  u_alpha/1 -> Mux5/1, Sum4/1
  u_beta/1 -> Mux5/2, Sum5/1
  Divide1/1 -> Mux3/1, Divide/1
  Divide2/1 -> Mux3/2, Divide3/1
  w/1 -> Mux/1, Mux1/1
  Mux/1 -> Rz4/1
  Fcn/1 -> Sum4/2, izio6/2, Mux2/1
  Fcn1/1 -> Mux2/2, Sum5/2
  Mux1/1 -> Rz3/1
  Divide4/1 -> Memory1/1
  Subsystem/3(Lalpha_beta) -> Divide4/1, Divide5/1
  Integrator5/1 -> Rz2/1, izio/2, ibeta/1
  Divide5/1 -> Memory/1
  Mux2/1 -> izio2/1
  Mux3/1 -> izio3/1
  Mux4/1 -> izio7/3, izio1/1
  Memory/1 -> Sum5/4
  Memory1/1 -> izio5/1, Sum4/4, Sum1/2
  Rz3/1 -> Fcn1/1
  Rz4/1 -> Fcn/1
  Divide6/1 -> Sum1/1
  Sum1/1 -> izio6/1
  Rz5/1 -> izio7/1
  Mux5/1 -> izio7/2

== system MyModel_Close_v1/Subsystem/Subsystem/dq-sixphasePMSM/dynamics/Theta Generator (-pi, pi) ==
  pi : Inport
  In : Inport  Port=2
  Compare To Constant : simulink/Logic and Bit Operations/Compare To Constant  relop=>  const=pi/2  OutDataTypeStr=uint8  ZeroCross=off
  Constant3 : Constant  Value=0
  Sum2 : Sum  Inputs=+-
  Switch : Switch  Threshold=0.5
  Out : Outport
  wires:
  Compare To Constant/1 -> Switch/2
  Switch/1 -> Sum2/2
  Constant3/1 -> Switch/3
  pi/1 -> Switch/1
  In/1 -> Sum2/1, Compare To Constant/1
  Sum2/1 -> Out/1

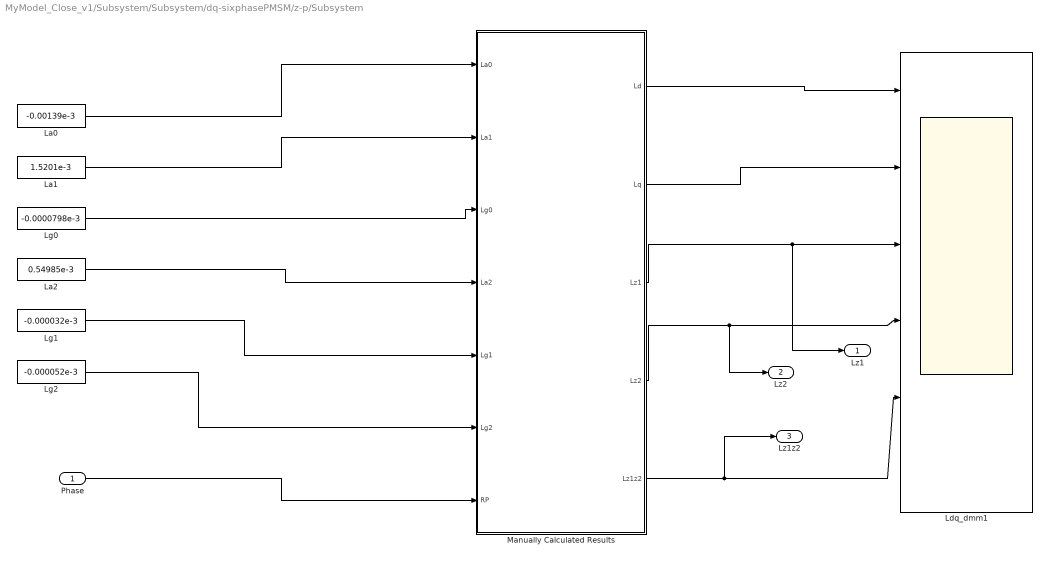
== system MyModel_Close_v1/Subsystem/Subsystem/dq-sixphasePMSM/z-p/Subsystem ==
  Phase : Inport
  La0 : Constant  Value=-0.00139e-3
  La1 : Constant  Value=1.5201e-3
  La2 : Constant  Value=0.54985e-3
  Ldq_dmm1 : Scope  NumInputPorts=6
  Lg0 : Constant  Value=-0.0000798e-3
  Lg1 : Constant  Value=-0.000032e-3
  Lg2 : Constant  Value=-0.000052e-3
  "Manually Calculated Results " : MATLAB Function  TreatAsAtomicUnit=on
  Lz1 : Outport
  Lz2 : Outport  Port=2
  Lz1z2 : Outport  Port=3
  wires:
  "Manually Calculated Results "/3(Lz1) -> Lz1/1, Ldq_dmm1/3
  Lg2/1 -> "Manually Calculated Results "/6(Lg2)
  Lg1/1 -> "Manually Calculated Results "/5(Lg1)
  "Manually Calculated Results "/2(Lq) -> Ldq_dmm1/2
  Lg0/1 -> "Manually Calculated Results "/3(Lg0)
  "Manually Calculated Results "/4(Lz2) -> Lz2/1, Ldq_dmm1/4
  "Manually Calculated Results "/1(Ld) -> Ldq_dmm1/1
  "Manually Calculated Results "/5(Lz1z2) -> Lz1z2/1, Ldq_dmm1/5
  La0/1 -> "Manually Calculated Results "/1(La0)
  La1/1 -> "Manually Calculated Results "/2(La1)
  La2/1 -> "Manually Calculated Results "/4(La2)
  Phase/1 -> "Manually Calculated Results "/7(RP)

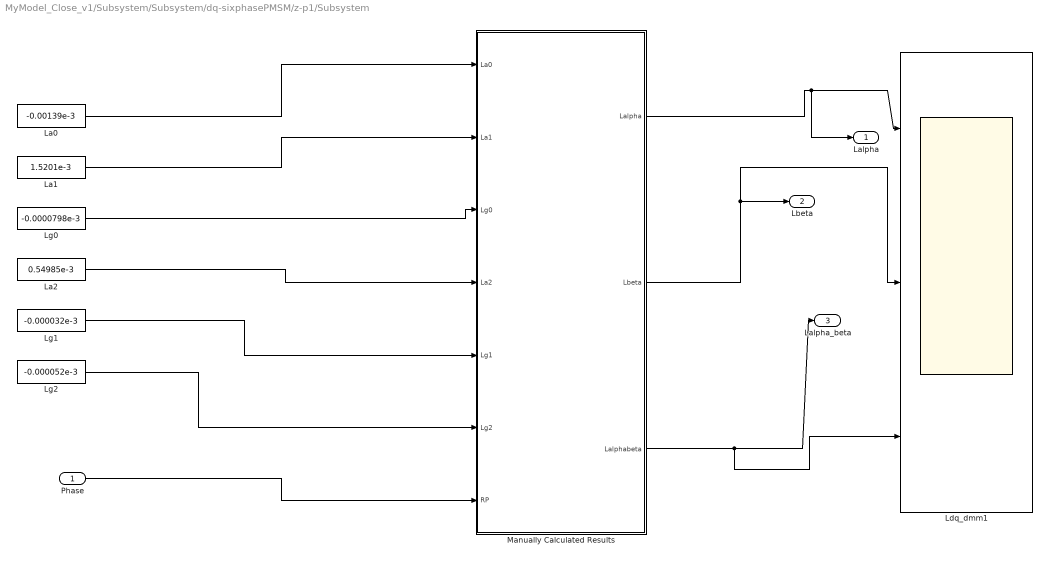
== system MyModel_Close_v1/Subsystem/Subsystem/dq-sixphasePMSM/z-p1/Subsystem ==
  Phase : Inport
  La0 : Constant  Value=-0.00139e-3
  La1 : Constant  Value=1.5201e-3
  La2 : Constant  Value=0.54985e-3
  Ldq_dmm1 : Scope  NumInputPorts=3
  Lg0 : Constant  Value=-0.0000798e-3
  Lg1 : Constant  Value=-0.000032e-3
  Lg2 : Constant  Value=-0.000052e-3
  "Manually Calculated Results " : MATLAB Function  TreatAsAtomicUnit=on
  Lalpha : Outport
  Lbeta : Outport  Port=2
  Lalpha_beta : Outport  Port=3
  wires:
  Lg2/1 -> "Manually Calculated Results "/6(Lg2)
  Lg1/1 -> "Manually Calculated Results "/5(Lg1)
  "Manually Calculated Results "/2(Lbeta) -> Ldq_dmm1/2, Lbeta/1
  Lg0/1 -> "Manually Calculated Results "/3(Lg0)
  "Manually Calculated Results "/1(Lalpha) -> Lalpha/1, Ldq_dmm1/1
  La0/1 -> "Manually Calculated Results "/1(La0)
  La1/1 -> "Manually Calculated Results "/2(La1)
  La2/1 -> "Manually Calculated Results "/4(La2)
  Phase/1 -> "Manually Calculated Results "/7(RP)
  "Manually Calculated Results "/3(Lalphabeta) -> Ldq_dmm1/3, Lalpha_beta/1

== matlab function MyModel_Close_v1/Subsystem/clark1 ==
  data: falpha output; fa input; fbeta output; fb input; fc input; fd input; fe input; fx output; fy output; fo1 output; fo2 output; ff input
function [falpha,fbeta,fx,fy,fo1,fo2] = clark(fa,fb,fc,fd,fe,ff)

T=1/sqrt(3)*[1,  (-1/2),    (-1/2),       sqrt(3)/2,  -sqrt(3)/2,  0;
       0,  sqrt(3)/2, (-sqrt(3)/2), 1/2,        1/2,        -1;
       1,  (-1/2),    (-1/2),       -sqrt(3)/2, sqrt(3)/2,   0;
       0,  -sqrt(3)/2,sqrt(3)/2,    1/2,        1/2,        -1;
       1,  1,         1,            0,          0,           0;
       0,  0,         0,            1,          1,           1];
X=[fa;fb;fc;fd;fe;ff];
Y=T*X;
falpha=Y(1);
fbeta=Y(2);
fx=Y(3);
fy=Y(4);
fo1=Y(5);
fo2=Y(6);
end

== matlab function MyModel_Close_v1/Subsystem/Embedded MATLAB Function ==
  data: uo output; uab input; ua output; ubc input; ucd input; ude input; uef input; ub output; uc output; ud output; ue output; uf output
function [uo,ua,ub,uc,ud,ue,uf] = fcn(uab,ubc,ucd,ude,uef)

%#codegen
uxx = [uab,ubc,ucd,ude,uef,0,0]';
T = [0 1 -1 0 0 0 0;
     0 0 1 -1 0 0 0;
     1 0 0 1 -1 0 0;
     0 0 0 0 1 -1 0;
     0 0 0 0 0 1 -1;
     0 1 1 1 0 0 0;
     0 0 0 0 1 1 1];
I = T \ uxx;
uo = I(1);
ua = I(2);
ub = I(3);
uc = I(4);
ud = I(5);
ue = I(6);
uf = I(7);

== matlab function MyModel_Close_v1/Subsystem/Subsystem/dq-sixphasePMSM/Embedded MATLAB Function1 ==
  data: ualpha output; ua input; ub input; uc input; ud input; ue input; uf input; ubeta output
function [ualpha,ubeta] = fcn(ua,ub,uc,ud,ue,uf)

%#eml
uxx=[ua,ub,uc,ud,ue,uf]';
T=1/sqrt(3)*[1 sqrt(3)/2 -1/2 -sqrt(3)/2 -1/2 0;
    0 1/2 sqrt(3)/2 1/2 -sqrt(3)/2 -1;
    1 -sqrt(3)/2 -1/2 sqrt(3)/2 -1/2 0;
    0 1/2 -sqrt(3)/2 1/2 sqrt(3)/2 -1;
    1 0 1 0 1 0;
    0 1 0 1 0 1];
I=T*uxx;
ualpha=I(1);
ubeta=I(2);

== matlab function MyModel_Close_v1/Subsystem/Subsystem/dq-sixphasePMSM/Embedded MATLAB Function2 ==
  data: ia output; ialpha input; ibeta input; iz1 input; iz2 input; iz3 input; iz4 input; ib output; ic output; id output; ie output; if1 output
function [ia,ib,ic,id,ie,if1] = fcn(ialpha,ibeta,iz1,iz2,iz3,iz4)

%#eml
uxx=[ialpha,ibeta,iz1,iz2,iz3,iz4]';
T=1/sqrt(3)*[1 sqrt(3)/2 -1/2 -sqrt(3)/2 -1/2 0;
    0 1/2 sqrt(3)/2 1/2 -sqrt(3)/2 -1;
    1 -sqrt(3)/2 -1/2 sqrt(3)/2 -1/2 0;
    0 1/2 -sqrt(3)/2 1/2 sqrt(3)/2 -1;
    1 0 1 0 1 0;
    0 1 0 1 0 1];
I=inv(T)*uxx;
ia=I(1);
ib=I(2);
ic=I(3);
id=I(4);
ie=I(5);
if1=I(6);

== matlab function MyModel_Close_v1/Subsystem/Subsystem/dq-sixphasePMSM/Embedded MATLAB Function3 ==
  data: ialpha input; id output; iq output; ibeta input; theta input
function [id,iq] = fcn(ialpha,ibeta,theta)

%#eml
uxx=[ialpha,ibeta]';
T=[cos(theta),-sin(theta);sin(theta),cos(theta)];
I=inv(T)*uxx;
id=I(1);
iq=I(2);

== matlab function MyModel_Close_v1/Subsystem/Subsystem/dq-sixphasePMSM/z-p/Subsystem/Manually Calculated Results  ==
  data: La0 input; Ld output; La1 input; Lg0 input; La2 input; Lg1 input; Lg2 input; RP input; Lq output; Lz1 output; Lz2 output; Lz1z2 output
function [Ld,Lq,Lz1,Lz2,Lz1z2] = fcn(La0,La1,Lg0,La2,Lg1,Lg2,RP)
%#codegen
Ld=3*La0+La1+sqrt(3)*La2+40*(1/2*Lg0+Lg1+Lg2);
Lq=3*La0+sqrt(3)*La2+La1-40*(1/2*Lg0+Lg1+Lg2);
Lz1=La1+cos(2*RP)*40*(1/2*Lg0-Lg1+Lg2)-sqrt(3)*La2;
Lz2=La1-cos(2*RP)*40*(1/2*Lg0-Lg1+Lg2)-sqrt(3)*La2;
Lz1z2=-sin(2*RP)*40*(1/2*Lg0-Lg1+Lg2);

== matlab function MyModel_Close_v1/Subsystem/Subsystem/dq-sixphasePMSM/z-p1/Subsystem/Manually Calculated Results  ==
  data: La0 input; Lalpha output; La1 input; Lg0 input; La2 input; Lg1 input; Lg2 input; RP input; Lbeta output; Lalphabeta output
function [Lalpha,Lbeta,Lalphabeta] = fcn(La0,La1,Lg0,La2,Lg1,Lg2,RP)
%#codegen
Lalpha=3*La0+La1+sqrt(3)*La2+40*(1/2*Lg0+Lg1+Lg2)*cos(2*RP);
Lbeta=3*La0+sqrt(3)*La2+La1-40*(1/2*Lg0+Lg1+Lg2)*cos(2*RP);
Lalphabeta=40*(1/2*Lg0+Lg1+Lg2)*sin(2*RP);

== matlab function MyModel_Close_v1/SVPWM3/Embedded MATLAB Function2 ==
  data: N input; T1 output; Ualpha input; Ubeta input; Tpwm input; T2 output; T3 output; T4 output; T0 output; udc input; Ux input; Uy input
function [T1, T2, T3, T4, T0] = fcn(N, Ualpha, Ubeta, Tpwm, udc, Ux,Uy)

m=sqrt(3)/2+1/2*1i;

%等功率clarke反变换
ab44=1/sqrt(3)*udc*[1,m^4,m^8,m,m^5,m^9]*[1;0;0;1;0;0];
xy44=1/sqrt(3)*udc*[1,m^8,m^4,m^5,m,m^9]*[1;0;0;1;0;0];

ab64=1/sqrt(3)*udc*[1,m^4,m^8,m,m^5,m^9]*[1;1;0;1;0;0];
xy64=1/sqrt(3)*udc*[1,m^8,m^4,m^5,m,m^9]*[1;1;0;1;0;0];
        
ab66=1/sqrt(3)*udc*[1,m^4,m^8,m,m^5,m^9]*[1;1;0;1;1;0];
xy66=1/sqrt(3)*udc*[1,m^8,m^4,m^5,m,m^9]*[1;1;0;1;1;0];

ab26=1/sqrt(3)*udc*[1,m^4,m^8,m,m^5,m^9]*[0;1;0;1;1;0];
xy26=1/sqrt(3)*udc*[1,m^8,m^4,m^5,m,m^9]*[0;1;0;1;1;0];

ab22=1/sqrt(3)*udc*[1,m^4,m^8,m,m^5,m^9]*[0;1;0;0;1;0];
xy22=1/sqrt(3)*udc*[1,m^8,m^4,m^5,m,m^9]*[0;1;0;0;1;0];

ab32=1/sqrt(3)*udc*[1,m^4,m^8,m,m^5,m^9]*[0;1;1;0;1;0];
xy32=1/sqrt(3)*udc*[1,m^8,m^4,m^5,m,m^9]*[0;1;1;0;1;0];

ab33=1/sqrt(3)*udc*[1,m^4,m^8,m,m^5,m^9]*[0;1;1;0;1;1];
xy33=1/sqrt(3)*udc*[1,m^8,m^4,m^5,m,m^9]*[0;1;1;0;1;1];

ab13=1/sqrt(3)*udc*[1,m^4,m^8,m,m^5,m^9]*[0;0;1;0;1;1];
xy13=1/sqrt(3)*udc*[1,m^8,m^4,m^5,m,m^9]*[0;0;1;0;1;1];

ab11=1/sqrt(3)*udc*[1,m^4,m^8,m,m^5,m^9]*[0;0;1;0;0;1];
xy11=1/sqrt(3)*udc*[1,m^8,m^4,m^5,m,m^9]*[0;0;1;0;0;1];

ab51=1/sqrt(3)*udc*[1,m^4,m^8,m,m^5,m^9]*[1;0;1;0;0;1];
xy51=1/sqrt(3)*udc*[1,m^8,m^4,m^5,m,m^9]*[1;0;1;0;0;1];

ab55=1/sqrt(3)*udc*[1,m^4,m^8,m,m^5,m^9]*[1;0;1;1;0;1];
xy55=1/sqrt(3)*udc*[1,m^8,m^4,m^5,m,m^9]*[1;0;1;1;0;1];

ab45=1/sqrt(3)*udc*[1,m^4,m^8,m,m^5,m^9]*[1;0;0;1;0;1];
xy45=1/sqrt(3)*udc*[1,m^8,m^4,m^5,m,m^9]*[1;0;0;1;0;1];

switch N
    case 1
        X=[real(ab55),real(ab45),real(ab44),real(ab64);
           imag(ab55),imag(ab45),imag(ab44),imag(ab64);
           real(xy55),real(xy45),real(xy44),real(xy64);
           imag(xy55),imag(xy45),imag(xy44),imag(xy64)];

    case 2
        X=[real(ab45),real(ab44),real(ab64),real(ab66);
           imag(ab45),imag(ab44),imag(ab64),imag(ab66);
           real(xy45),real(xy44),real(xy64),real(xy66);
           imag(xy45),imag(xy44),imag(xy64),imag(xy66)];

    case 3
        X=[real(ab44),real(ab64),real(ab66),real(ab26);
           imag(ab44),imag(ab64),imag(ab66),imag(ab26);
           real(xy44),real(xy64),real(xy66),real(xy26);
           imag(xy44),imag(xy64),imag(xy66),imag(xy26)];

    case 4
        X=[real(ab64),real(ab66),real(ab26),real(ab22);
           imag(ab64),imag(ab66),imag(ab26),imag(ab22);
           real(xy64),real(xy66),real(xy26),real(xy22);
           imag(xy64),imag(xy66),imag(xy26),imag(xy22)];

    case 5
        X=[real(ab66),real(ab26),real(ab22),real(ab32);
           imag(ab66),imag(ab26),imag(ab22),imag(ab32);
           real(xy66),real(xy26),real(xy22),real(xy32);
           imag(xy66),imag(xy26),imag(xy22),imag(xy32)];

    case 6
        X=[real(ab26),real(ab22),real(ab32),real(ab33);
           imag(ab26),imag(ab22),imag(ab32),imag(ab33);
           real(xy26),real(xy22),real(xy32),real(xy33);
           imag(xy26),imag(xy22),imag(xy32),imag(xy33)];

    case 7
        X=[real(ab22),real(ab32),real(ab33),real(ab13);
           imag(ab22),imag(ab32),imag(ab33),imag(ab13);
           real(xy22),real(xy32),real(xy33),real(xy13);
           imag(xy22),imag(xy32),imag(xy33),imag(xy13)];

    case 8
        X=[real(ab32),real(ab33),real(ab13),real(ab11);
           imag(ab32),imag(ab33),imag(ab13),imag(ab11);
           real(xy32),real(xy33),real(xy13),real(xy11);
           imag(xy32),imag(xy33),imag(xy13),imag(xy11)];

    case 9
        X=[real(ab33),real(ab13),real(ab11),real(ab51);
           imag(ab33),imag(ab13),imag(ab11),imag(ab51);
           real(xy33),real(xy13),real(xy11),real(xy51);
           imag(xy33),imag(xy13),imag(xy11),imag(xy51)];

    case 10
        X=[real(ab13),real(ab11),real(ab51),real(ab55);
           imag(ab13),imag(ab11),imag(ab51),imag(ab55);
           real(xy13),real(xy11),real(xy51),real(xy55);
           imag(xy13),imag(xy11),imag(xy51),imag(xy55)];

    case 11
        X=[real(ab11),real(ab51),real(ab55),real(ab45);
           imag(ab11),imag(ab51),imag(ab55),imag(ab45);
           real(xy11),real(xy51),real(xy55),real(xy45);
           imag(xy11),imag(xy51),imag(xy55),imag(xy45)];

    case 12
        X=[real(ab51),real(ab55),real(ab45),real(ab44);
           imag(ab51),imag(ab55),imag(ab45),imag(ab44);
           real(xy51),real(xy55),real(xy45),real(xy44);
           imag(xy51),imag(xy55),imag(xy45),imag(xy44)];

    otherwise
        X=[0,0,0,0;
           0,0,0,0;
           0,0,0,0;
           0,0,0,0];

end
Y=[Ualpha;Ubeta;Ux;Uy]*Tpwm;
T = X \ Y;

T1=T(1);
if T1<15e-6
    T1=15e-6;
end 
T2=T(2);
if T2<15e-6
    T2=15e-6;
end 
T3=T(3);
if T3<1e-6
    T3=1e-6;
end 
T4=T(4);
if T4<1e-6
    T4=1e-6;
end

% T1=T(1);
% T2=T(2);
% T3=T(3);
% T4=T(4);

Tsum=T1+T2+T3+T4;
if Tsum>Tpwm
    T1=T1*Tpwm/Tsum;
    T2=T2*Tpwm/Tsum;
    T3=T3*Tpwm/Tsum;
    T4=T4*Tpwm/Tsum;
end
T0=Tpwm-T1-T2-T3-T4;
end

== matlab function MyModel_Close_v1/SVPWM3/Embedded MATLAB Function6 ==
  data: N output; ualfa input; ubeta input; TH output
function [N,TH] = fcn(ualfa,ubeta)

%#xsxx
[TH,R] = cart2pol(ualfa,ubeta);
if TH<0
    TH=TH+2*pi;
end
N=floor((TH+pi/12)/(pi/6))+1;
if N==13
    N=1;
end;

== matlab function MyModel_Close_v1/SVPWM3/rest of others ==
  data: N input; T1 input; T2 input; T3 input; T4 input; T0 input; a1 output; a2 output; b1 output; b2 output; c1 output; c2 output; d1 output; d2 output; e1 output; e2 output; f1 output; f2 output
function [a1,a2,b1,b2,c1,c2,d1,d2,e1,e2,f1,f2] = fcn(N,T1,T2,T3,T4,T0)

%#xsxx
Ta=T0/4;
Tb=Ta+T2;
Tc=Tb+T1;
Td=Tc+T0/2;
Te=Td+T4;
Tf=Te+T3;

Ta1=T0/4;
Tb1=Ta1+T1;
Tc1=Tb1+T2;
Td1=Tc1+T0/2;
Te1=Td1+T3;
Tf1=Te1+T4;

%a1:phase A CMPA
%a2:phase A CMPB

a1 = 0;
a2 = 0;
b1 = 0;
b2 = 0;
c1 = 0;
c2 = 0;
d1 = 0;
d2 = 0;
e1 = 0;
e2 = 0;
f1 = 0;
f2 = 0;

if N==1
    a1=Ta;%TIme of "00" voltage vector 
    a2=Tf;%TIme of "48" voltage vector 
    d1=Ta;
    d2=Tf;
    b1=Tc;%TIme of "51" voltage vector 
    b2=Te;%TIme of "56" voltage vector 
    e1=Tc;
    e2=Td;
    c1=Tb;%TIme of "49" voltage vector 
    c2=Td;%TIme of "63" voltage vector 
    f1=Ta;
    f2=Td;
elseif N==2
    a1=Ta;
    a2=Tf;
    d1=Ta;
    d2=Tf;
    b1=Tc;
    b2=Tf;
    e1=Tc;
    e2=Te;
    c1=Tc;
    c2=Td;
    f1=Tb;
    f2=Td;
elseif N==3
    a1=Ta1;
    a2=Te1;
    d1=Ta1;
    d2=Tf1;
    b1=Tb1;
    b2=Tf1;
    e1=Tc1;
    e2=Tf1;
    c1=Tc1;
    c2=Td1;
    f1=Tc1;
    f2=Td1;
elseif N==4
    a1=Ta1;
    a2=Td1;
    d1=Ta1;
    d2=Te1;
    b1=Ta1;
    b2=Tf1;
    e1=Tb1;
    e2=Tf1;
    c1=Tc1;
    c2=Td1;
    f1=Tc1;
    f2=Td1;
elseif N==5
    a1=Tb;
    a2=Td;
    d1=Ta;
    d2=Td;
    b1=Ta;
    b2=Tf;
    e1=Ta;
    e2=Tf;
    c1=Tc;
    c2=Te;
    f1=Tc;
    f2=Td;
elseif N==6
    a1=Tc;
    a2=Td;
    d1=Tb;
    d2=Td;
    b1=Ta;
    b2=Tf;
    e1=Ta;
    e2=Tf;
    c1=Tc;
    c2=Tf;
    f1=Tc;
    f2=Te;
elseif N==7
    a1=Tc1;
    a2=Td1;
    d1=Tc1;
    d2=Td1;
    b1=Ta1;
    b2=Te1;
    e1=Ta1;
    e2=Tf1;
    c1=Tb1;
    c2=Tf1;
    f1=Tc1;
    f2=Tf1;
elseif N==8
    a1=Tc1;
    a2=Td1;
    d1=Tc1;
    d2=Td1;
    b1=Ta1;
    b2=Td1;
    e1=Ta1;
    e2=Te1;
    c1=Ta1;
    c2=Tf1;
    f1=Tb1;
    f2=Tf1;
elseif N==9
    a1=Tc;
    a2=Te;
    d1=Tc;
    d2=Td;
    b1=Tb;
    b2=Td;
    e1=Ta;
    e2=Td;
    c1=Ta;
    c2=Tf;
    f1=Ta;
    f2=Tf;
elseif N==10
    a1=Tc;
    a2=Tf;
    d1=Tc;
    d2=Te;
    b1=Tc;
    b2=Td;
    e1=Tb;
    e2=Td;
    c1=Ta;
    c2=Tf;
    f1=Ta;
    f2=Tf;
elseif N==11
    a1=Tb1;
    a2=Tf1;
    d1=Tc1;
    d2=Tf1;
    b1=Tc1;
    b2=Td1;
    e1=Tc1;
    e2=Td1;
    c1=Ta1;
    c2=Te1;
    f1=Ta1;
    f2=Tf1;
elseif N==12
    a1=Ta1;
    a2=Tf1;
    d1=Tb1;
    d2=Tf1;
    b1=Tc1;
    b2=Td1;
    e1=Tc1;
    e2=Td1;
    c1=Ta1;
    c2=Td1;
    f1=Ta1;
    f2=Te1;
end
